simulink model "EGRVlv_DDSens"  (R2018a)
settings: configuration reference "cs_ert" (kept outside this file)
model workspace (MAT data in the model file):
  EGRVlv_DDSens_DT = 10
values from neighbouring files (symbols this model uses):
  EGRVlv_rAdapDiffPlausLgT_C = 20.0    [EGRVlv_DDSens.sldd]
  EGRVlv_rTransf_CUR : value not decoded    [EGRVlv_DDSens.sldd]
  EGRVlv_rTransf_CURX : value not decoded    [EGRVlv_DDSens.sldd]
  EGRVlv_tiMaxDefDeb_C = 200.0    [EGRVlv_DDSens.sldd]
  EGRVlv_tiMaxOKDeb_C = 200.0    [EGRVlv_DDSens.sldd]
  EGRVlv_tiMinDefDeb_C = 200.0    [EGRVlv_DDSens.sldd]
  EGRVlv_tiMinOKDeb_C = 200.0    [EGRVlv_DDSens.sldd]
  EGRVlv_tiPhysRngHiDefDeb_C = 200.0    [EGRVlv_DDSens.sldd]
  EGRVlv_tiPhysRngHiOKDeb_C = 200.0    [EGRVlv_DDSens.sldd]
  EGRVlv_tiPhysRngLoDefDeb_C = 200.0    [EGRVlv_DDSens.sldd]
  EGRVlv_tiPhysRngLoOKDeb_C = 200.0    [EGRVlv_DDSens.sldd]
  EGRVlv_uSRCMax_C = 4800.0    [EGRVlv_DDSens.sldd]
  EGRVlv_uSRCMin_C = 200.0    [EGRVlv_DDSens.sldd]
undefined symbols (not defined in the file or in its folder): CEngDsT_tTransf_CURX
libraries: sllib x4
settings Model: DataDictionary=EGRVlv_DDSens.sldd  Creator=zhoutinglin  LastModifiedBy=zhoutinglin

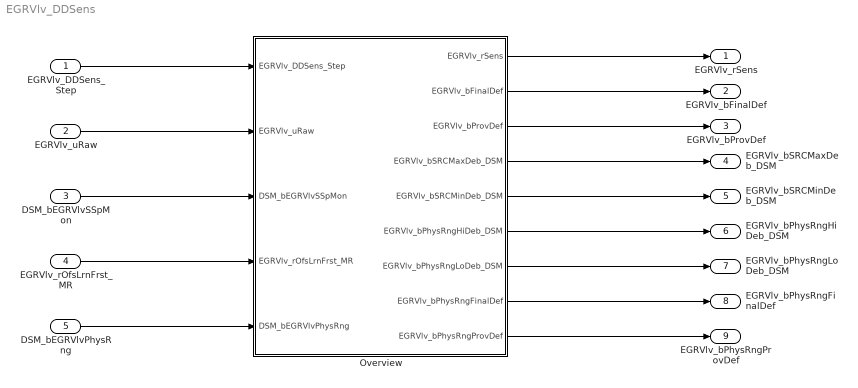
== system EGRVlv_DDSens ==
  EGRVlv_DDSens_Step : Inport  OutputFunctionCall=on
  EGRVlv_uRaw : Inport  Description=Raw voltage value of position sensor  Port=2  OutMin=0  OutMax=5000  OutDataTypeStr=Volt_mV  Unit=mv  PortDimensions=[1 1]
  DSM_bEGRVlvSSpMon : Inport  Description=Status of FId_EGRVlvSSpMon  Port=3  OutMin=0  OutMax=1  OutDataTypeStr=boolean  PortDimensions=[1 1]
  EGRVlv_rOfsLrnFrst_MR : Inport  Description=First learnt offset value read from EEPROM  Port=4  OutMin=-100  OutMax=100  OutDataTypeStr=DutyCycle  Unit=%  PortDimensions=[1 1]
  DSM_bEGRVlvPhysRng : Inport  Description=Status of FId_EGRVlvPhysRng  Port=5  OutMin=0  OutMax=1  OutDataTypeStr=boolean  PortDimensions=[1 1]
  Overview : Subsystem
  EGRVlv_rSens : Outport  Description=Sensed value of actuator position without error handling  OutMin=-100  OutMax=100  OutDataTypeStr=DutyCycle  Unit=%  PortDimensions=[1 1]
  EGRVlv_bFinalDef : Outport  Description=the final fault flag  Port=2  OutMin=0  OutMax=1  OutDataTypeStr=boolean  PortDimensions=[1 1]
  EGRVlv_bProvDef : Outport  Description=the fault flag for the moment  Port=3  OutMin=0  OutMax=1  OutDataTypeStr=boolean  PortDimensions=[1 1]
  EGRVlv_bSRCMaxDeb_DSM : Outport  Description=SRC High for EGR position sensor voltage  Port=4  OutMin=0  OutMax=1  OutDataTypeStr=boolean  PortDimensions=[1 1]
  EGRVlv_bSRCMinDeb_DSM : Outport  Description=SRC Low for EGR position sensor voltage  Port=5  OutMin=0  OutMax=1  OutDataTypeStr=boolean  PortDimensions=[1 1]
  EGRVlv_bPhysRngHiDeb_DSM : Outport  Description=Status of EGRVlv_bPhysRngHiDeb  Port=6  OutMin=0  OutMax=1  OutDataTypeStr=boolean  PortDimensions=[1 1]
  EGRVlv_bPhysRngLoDeb_DSM : Outport  Description=Status of EGRVlv_bPhysRngLoDeb  Port=7  OutMin=0  OutMax=1  OutDataTypeStr=boolean  PortDimensions=[1 1]
  EGRVlv_bPhysRngFinalDef : Outport  Description=Status Sensor of the EGR valve physical Signal range check finally defect  Port=8  OutMin=0  OutMax=1  OutDataTypeStr=boolean  PortDimensions=[1 1]
  EGRVlv_bPhysRngProvDef : Outport  Description=Status Sensor of the EGR valve physical Signal range check temporary defect  Port=9  OutMin=0  OutMax=1  OutDataTypeStr=boolean  PortDimensions=[1 1]
  wires:
  EGRVlv_DDSens_Step/1 -> Overview/1(EGRVlv_DDSens_Step)
  EGRVlv_uRaw/1 -> Overview/2(EGRVlv_uRaw)
  DSM_bEGRVlvSSpMon/1 -> Overview/3(DSM_bEGRVlvSSpMon)
  EGRVlv_rOfsLrnFrst_MR/1 -> Overview/4(EGRVlv_rOfsLrnFrst_MR)
  DSM_bEGRVlvPhysRng/1 -> Overview/5(DSM_bEGRVlvPhysRng)
  Overview/1(EGRVlv_rSens) -> EGRVlv_rSens/1
  Overview/2(EGRVlv_bFinalDef) -> EGRVlv_bFinalDef/1
  Overview/3(EGRVlv_bProvDef) -> EGRVlv_bProvDef/1
  Overview/4(EGRVlv_bSRCMaxDeb_DSM) -> EGRVlv_bSRCMaxDeb_DSM/1
  Overview/5(EGRVlv_bSRCMinDeb_DSM) -> EGRVlv_bSRCMinDeb_DSM/1
  Overview/6(EGRVlv_bPhysRngHiDeb_DSM) -> EGRVlv_bPhysRngHiDeb_DSM/1
  Overview/7(EGRVlv_bPhysRngLoDeb_DSM) -> EGRVlv_bPhysRngLoDeb_DSM/1
  Overview/8(EGRVlv_bPhysRngFinalDef) -> EGRVlv_bPhysRngFinalDef/1
  Overview/9(EGRVlv_bPhysRngProvDef) -> EGRVlv_bPhysRngProvDef/1

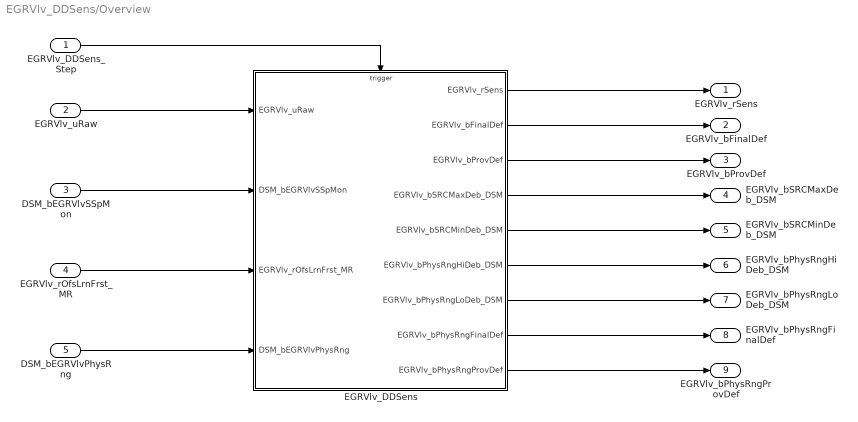
== system EGRVlv_DDSens/Overview ==
  EGRVlv_DDSens_Step : Inport
  EGRVlv_uRaw : Inport  Port=2
  DSM_bEGRVlvSSpMon : Inport  Port=3
  EGRVlv_rOfsLrnFrst_MR : Inport  Port=4
  DSM_bEGRVlvPhysRng : Inport  Port=5
  EGRVlv_DDSens : Subsystem
  EGRVlv_rSens : Outport
  EGRVlv_bFinalDef : Outport  Port=2
  EGRVlv_bProvDef : Outport  Port=3
  EGRVlv_bSRCMaxDeb_DSM : Outport  Port=4
  EGRVlv_bSRCMinDeb_DSM : Outport  Port=5
  EGRVlv_bPhysRngHiDeb_DSM : Outport  Port=6
  EGRVlv_bPhysRngLoDeb_DSM : Outport  Port=7
  EGRVlv_bPhysRngFinalDef : Outport  Port=8
  EGRVlv_bPhysRngProvDef : Outport  Port=9
  wires:
  EGRVlv_uRaw/1 -> EGRVlv_DDSens/1(EGRVlv_uRaw)
  DSM_bEGRVlvSSpMon/1 -> EGRVlv_DDSens/2(DSM_bEGRVlvSSpMon)
  EGRVlv_rOfsLrnFrst_MR/1 -> EGRVlv_DDSens/3(EGRVlv_rOfsLrnFrst_MR)
  DSM_bEGRVlvPhysRng/1 -> EGRVlv_DDSens/4(DSM_bEGRVlvPhysRng)
  EGRVlv_DDSens/1(EGRVlv_rSens) -> EGRVlv_rSens/1
  EGRVlv_DDSens/2(EGRVlv_bFinalDef) -> EGRVlv_bFinalDef/1
  EGRVlv_DDSens/3(EGRVlv_bProvDef) -> EGRVlv_bProvDef/1
  EGRVlv_DDSens/4(EGRVlv_bSRCMaxDeb_DSM) -> EGRVlv_bSRCMaxDeb_DSM/1
  EGRVlv_DDSens/5(EGRVlv_bSRCMinDeb_DSM) -> EGRVlv_bSRCMinDeb_DSM/1
  EGRVlv_DDSens/6(EGRVlv_bPhysRngHiDeb_DSM) -> EGRVlv_bPhysRngHiDeb_DSM/1
  EGRVlv_DDSens/7(EGRVlv_bPhysRngLoDeb_DSM) -> EGRVlv_bPhysRngLoDeb_DSM/1
  EGRVlv_DDSens/8(EGRVlv_bPhysRngFinalDef) -> EGRVlv_bPhysRngFinalDef/1
  EGRVlv_DDSens/9(EGRVlv_bPhysRngProvDef) -> EGRVlv_bPhysRngProvDef/1
  EGRVlv_DDSens_Step/1 -> EGRVlv_DDSens/Trigger

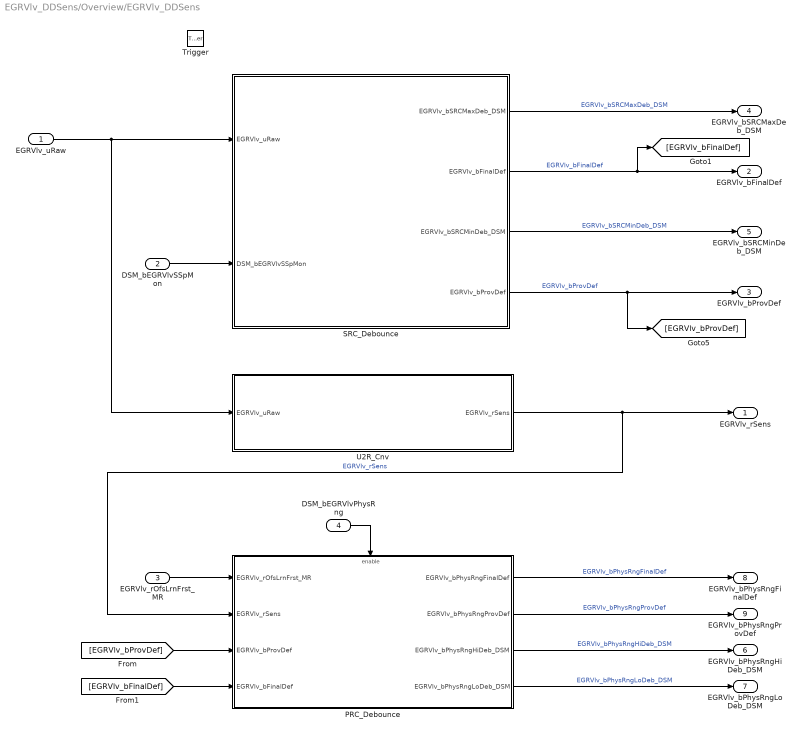
== system EGRVlv_DDSens/Overview/EGRVlv_DDSens ==
  EGRVlv_uRaw : Inport  Tag=mv
  DSM_bEGRVlvSSpMon : Inport  Port=2
  EGRVlv_rOfsLrnFrst_MR : Inport  Port=3
  DSM_bEGRVlvPhysRng : Inport  Port=4
  Trigger : TriggerPort  TriggerType=function-call  VariantControl=Variant  PortDimensions=1
  PRC_Debounce : Subsystem
  SRC_Debounce : Subsystem
  U2R_Cnv : Subsystem
  EGRVlv_rSens : Outport  Tag=%
  EGRVlv_bFinalDef : Outport  Port=2
  EGRVlv_bProvDef : Outport  Port=3
  EGRVlv_bSRCMaxDeb_DSM : Outport  Port=4
  EGRVlv_bSRCMinDeb_DSM : Outport  Port=5
  EGRVlv_bPhysRngHiDeb_DSM : Outport  Port=6
  EGRVlv_bPhysRngLoDeb_DSM : Outport  Port=7
  EGRVlv_bPhysRngFinalDef : Outport  Port=8
  EGRVlv_bPhysRngProvDef : Outport  Port=9
  wires:
  SRC_Debounce/2(EGRVlv_bFinalDef) -> EGRVlv_bFinalDef/1, [EGRVlv_bFinalDef]  "EGRVlv_bFinalDef"
  EGRVlv_uRaw/1 -> SRC_Debounce/1(EGRVlv_uRaw), U2R_Cnv/1(EGRVlv_uRaw)
  SRC_Debounce/4(EGRVlv_bProvDef) -> EGRVlv_bProvDef/1, [EGRVlv_bProvDef]  "EGRVlv_bProvDef"
  U2R_Cnv/1(EGRVlv_rSens) -> EGRVlv_rSens/1, PRC_Debounce/2(EGRVlv_rSens)  "EGRVlv_rSens"
  EGRVlv_rOfsLrnFrst_MR/1 -> PRC_Debounce/1(EGRVlv_rOfsLrnFrst_MR)
  [EGRVlv_bProvDef] -> PRC_Debounce/3(EGRVlv_bProvDef)
  [EGRVlv_bFinalDef] -> PRC_Debounce/4(EGRVlv_bFinalDef)
  DSM_bEGRVlvSSpMon/1 -> SRC_Debounce/2(DSM_bEGRVlvSSpMon)
  PRC_Debounce/1(EGRVlv_bPhysRngFinalDef) -> EGRVlv_bPhysRngFinalDef/1  "EGRVlv_bPhysRngFinalDef"
  PRC_Debounce/2(EGRVlv_bPhysRngProvDef) -> EGRVlv_bPhysRngProvDef/1  "EGRVlv_bPhysRngProvDef"
  PRC_Debounce/3(EGRVlv_bPhysRngHiDeb_DSM) -> EGRVlv_bPhysRngHiDeb_DSM/1  "EGRVlv_bPhysRngHiDeb_DSM"
  PRC_Debounce/4(EGRVlv_bPhysRngLoDeb_DSM) -> EGRVlv_bPhysRngLoDeb_DSM/1  "EGRVlv_bPhysRngLoDeb_DSM"
  SRC_Debounce/1(EGRVlv_bSRCMaxDeb_DSM) -> EGRVlv_bSRCMaxDeb_DSM/1  "EGRVlv_bSRCMaxDeb_DSM"
  SRC_Debounce/3(EGRVlv_bSRCMinDeb_DSM) -> EGRVlv_bSRCMinDeb_DSM/1  "EGRVlv_bSRCMinDeb_DSM"
  DSM_bEGRVlvPhysRng/1 -> PRC_Debounce/Enable

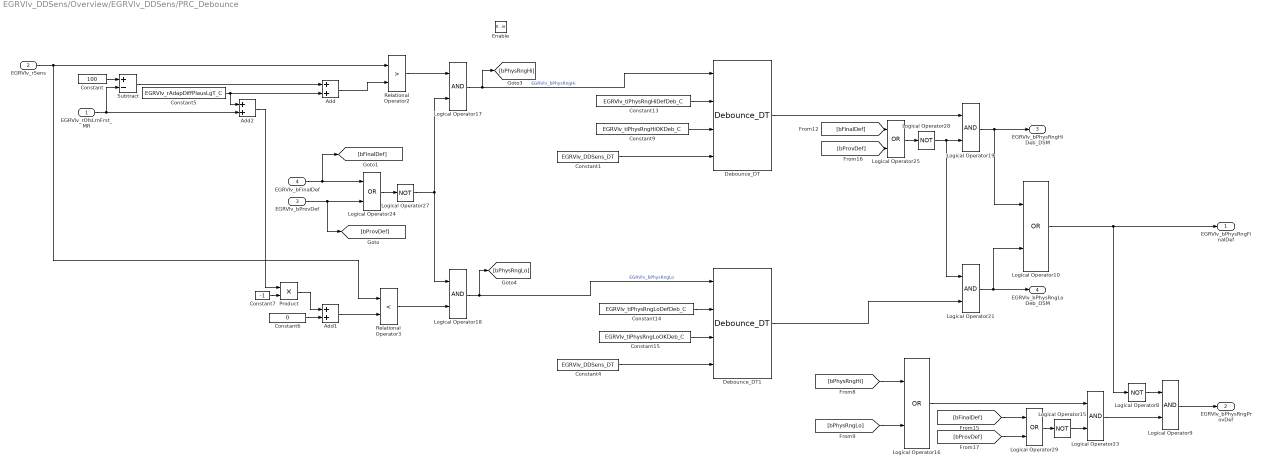
== system EGRVlv_DDSens/Overview/EGRVlv_DDSens/PRC_Debounce ==
  EGRVlv_rOfsLrnFrst_MR : Inport
  EGRVlv_rSens : Inport  Port=2
  EGRVlv_bProvDef : Inport  Port=3
  EGRVlv_bFinalDef : Inport  Port=4
  Enable : EnablePort
  Add : Sum  SaturateOnIntegerOverflow=on
  Add1 : Sum  SaturateOnIntegerOverflow=on  InputSameDT=on
  Add2 : Sum  SaturateOnIntegerOverflow=on
  Constant : Constant  Value=100  OutDataTypeStr=Inherit: Inherit via back propagation
  Constant1 : Constant  Value=EGRVlv_DDSens_DT  OutDataTypeStr=Inherit: Inherit via back propagation
  Constant13 : Constant  Value=EGRVlv_tiPhysRngHiDefDeb_C
  Constant14 : Constant  Value=EGRVlv_tiPhysRngLoDefDeb_C
  Constant15 : Constant  Value=EGRVlv_tiPhysRngLoOKDeb_C
  Constant4 : Constant  Value=EGRVlv_DDSens_DT  OutDataTypeStr=Inherit: Inherit via back propagation
  Constant5 : Constant  Value=EGRVlv_rAdapDiffPlausLgT_C
  Constant6 : Constant  Value=0  OutDataTypeStr=Inherit: Inherit via back propagation
  Constant7 : Constant  Value=-1  OutDataTypeStr=int8
  Constant9 : Constant  Value=EGRVlv_tiPhysRngHiOKDeb_C
  Debounce_DT : sllib/Debounce_DT
      settings: SourceProductName=sllib
  Debounce_DT1 : sllib/Debounce_DT
      settings: SourceProductName=sllib
  Logical Operator10 : Logic  Operator=OR  AllPortsSameDT=off  OutDataTypeStr=boolean
  Logical Operator{8,15,27..28} (4 alike) : Logic  Operator=NOT  AllPortsSameDT=off  OutDataTypeStr=boolean
  Logical Operator16 : Logic  Operator=OR  AllPortsSameDT=off  OutDataTypeStr=boolean
  Logical Operator{9,17..19,21,23} (6 alike) : Logic  AllPortsSameDT=off  OutDataTypeStr=boolean
  Logical Operator24 : Logic  Operator=OR  OutDataTypeStr=boolean
  Logical Operator25 : Logic  Operator=OR  OutDataTypeStr=boolean
  Logical Operator29 : Logic  Operator=OR  OutDataTypeStr=boolean
  Product : Product  OutDataTypeStr=Inherit: Inherit via back propagation  SaturateOnIntegerOverflow=on
  Relational Operator2 : RelationalOperator  Operator=>  OutDataTypeStr=boolean  RndMeth=Nearest  InputSameDT=on
  Relational Operator3 : RelationalOperator  Operator=<  OutDataTypeStr=boolean  RndMeth=Nearest  InputSameDT=on
  Subtract : Sum  Inputs=+-  SaturateOnIntegerOverflow=on
  EGRVlv_bPhysRngFinalDef : Outport  Tag=-  InitialOutput=0
  EGRVlv_bPhysRngProvDef : Outport  Tag=-  Port=2  InitialOutput=0
  EGRVlv_bPhysRngHiDeb_DSM : Outport  Tag=-  Port=3  InitialOutput=0
  EGRVlv_bPhysRngLoDeb_DSM : Outport  Tag=-  Port=4  InitialOutput=0
  wires:
  EGRVlv_rSens/1 -> Relational Operator2/1, Relational Operator3/1
  Constant15/1 -> Debounce_DT1/3
  Constant13/1 -> Debounce_DT/2
  Constant9/1 -> Debounce_DT/3
  Constant14/1 -> Debounce_DT1/2
  Constant1/1 -> Debounce_DT/4
  Constant4/1 -> Debounce_DT1/4
  Add/1 -> Relational Operator2/2
  Logical Operator17/1 -> Debounce_DT/1, [bPhysRngHi]  "EGRVlv_bPhysRngHi"
  Add1/1 -> Relational Operator3/2
  Logical Operator18/1 -> Debounce_DT1/1, [bPhysRngLo]  "EGRVlv_bPhysRngLo"
  Logical Operator19/1 -> Logical Operator10/1, EGRVlv_bPhysRngHiDeb_DSM/1
  Logical Operator21/1 -> EGRVlv_bPhysRngLoDeb_DSM/1, Logical Operator10/2
  [bPhysRngHi] -> Logical Operator16/1
  [bPhysRngLo] -> Logical Operator16/2
  Relational Operator2/1 -> Logical Operator17/1
  Logical Operator24/1 -> Logical Operator27/1
  Logical Operator25/1 -> Logical Operator28/1
  Logical Operator16/1 -> Logical Operator23/1
  Logical Operator15/1 -> Logical Operator23/2
  Relational Operator3/1 -> Logical Operator18/2
  EGRVlv_bFinalDef/1 -> [bFinalDef], Logical Operator24/1
  EGRVlv_bProvDef/1 -> Logical Operator24/2, [bProvDef]
  [bFinalDef] -> Logical Operator25/1
  [bProvDef] -> Logical Operator25/2
  Logical Operator27/1 -> Logical Operator17/2, Logical Operator18/1
  Logical Operator28/1 -> Logical Operator21/1, Logical Operator19/2
  [bFinalDef] -> Logical Operator29/1
  [bProvDef] -> Logical Operator29/2
  Logical Operator29/1 -> Logical Operator15/1
  Logical Operator10/1 -> EGRVlv_bPhysRngFinalDef/1, Logical Operator8/1
  Logical Operator8/1 -> Logical Operator9/1
  Logical Operator9/1 -> EGRVlv_bPhysRngProvDef/1
  Logical Operator23/1 -> Logical Operator9/2
  Constant/1 -> Subtract/1
  EGRVlv_rOfsLrnFrst_MR/1 -> Add2/2, Subtract/2
  Subtract/1 -> Add/1
  Constant5/1 -> Add/2, Add2/1
  Constant7/1 -> Product/2
  Constant6/1 -> Add1/2
  Product/1 -> Add1/1
  Add2/1 -> Product/1
  Debounce_DT/1 -> Logical Operator19/1
  Debounce_DT1/1 -> Logical Operator21/2

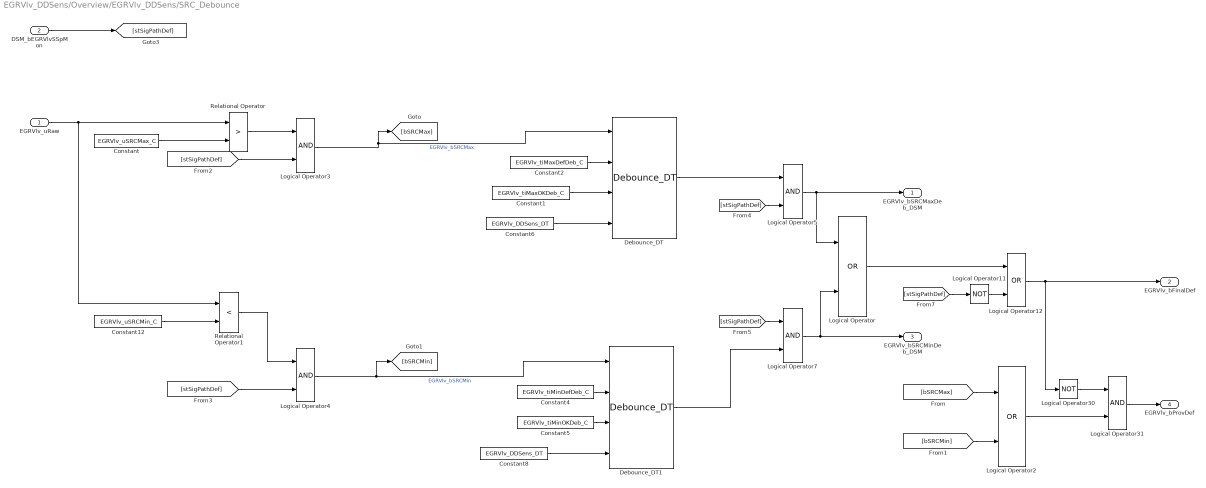
== system EGRVlv_DDSens/Overview/EGRVlv_DDSens/SRC_Debounce ==
  EGRVlv_uRaw : Inport  Tag=mv
  DSM_bEGRVlvSSpMon : Inport  Tag=-  Port=2
  Constant : Constant  Value=EGRVlv_uSRCMax_C
  Constant1 : Constant  Value=EGRVlv_tiMaxOKDeb_C
  Constant12 : Constant  Value=EGRVlv_uSRCMin_C
  Constant2 : Constant  Value=EGRVlv_tiMaxDefDeb_C
  Constant4 : Constant  Value=EGRVlv_tiMinDefDeb_C
  Constant5 : Constant  Value=EGRVlv_tiMinOKDeb_C
  Constant6 : Constant  Value=EGRVlv_DDSens_DT  OutDataTypeStr=Inherit: Inherit via back propagation
  Constant8 : Constant  Value=EGRVlv_DDSens_DT  OutDataTypeStr=Inherit: Inherit via back propagation
  Debounce_DT : sllib/Debounce_DT
      settings: SourceProductName=sllib
  Debounce_DT1 : sllib/Debounce_DT
      settings: SourceProductName=sllib
  Logical Operator : Logic  Operator=OR  AllPortsSameDT=off  OutDataTypeStr=boolean
  Logical Operator11 : Logic  Operator=NOT  AllPortsSameDT=off  OutDataTypeStr=boolean
  Logical Operator12 : Logic  Operator=OR  AllPortsSameDT=off  OutDataTypeStr=boolean
  Logical Operator2 : Logic  Operator=OR  AllPortsSameDT=off  OutDataTypeStr=boolean
  Logical Operator{3..5,7,31} (5 alike) : Logic  AllPortsSameDT=off  OutDataTypeStr=boolean
  Logical Operator30 : Logic  Operator=NOT  AllPortsSameDT=off  OutDataTypeStr=boolean
  Relational Operator : RelationalOperator  Operator=>  OutDataTypeStr=boolean  RndMeth=Nearest  InputSameDT=on
  Relational Operator1 : RelationalOperator  Operator=<  OutDataTypeStr=boolean  RndMeth=Nearest  InputSameDT=on
  EGRVlv_bSRCMaxDeb_DSM : Outport  Tag=-
  EGRVlv_bFinalDef : Outport  Tag=-  Port=2
  EGRVlv_bSRCMinDeb_DSM : Outport  Tag=-  Port=3
  EGRVlv_bProvDef : Outport  Tag=-  Port=4
  wires:
  Relational Operator1/1 -> Logical Operator4/1
  [stSigPathDef] -> Logical Operator4/2
  [stSigPathDef] -> Logical Operator5/2
  [stSigPathDef] -> Logical Operator7/1
  EGRVlv_uRaw/1 -> Relational Operator1/1, Relational Operator/1
  Logical Operator12/1 -> Logical Operator30/1, EGRVlv_bFinalDef/1
  Logical Operator30/1 -> Logical Operator31/1
  Logical Operator31/1 -> EGRVlv_bProvDef/1
  Logical Operator/1 -> Logical Operator12/1
  [stSigPathDef] -> Logical Operator11/1
  Logical Operator11/1 -> Logical Operator12/2
  Debounce_DT/1 -> Logical Operator5/1
  Constant4/1 -> Debounce_DT1/2
  Constant1/1 -> Debounce_DT/3
  Constant2/1 -> Debounce_DT/2
  Constant5/1 -> Debounce_DT1/3
  Constant6/1 -> Debounce_DT/4
  Constant8/1 -> Debounce_DT1/4
  Constant/1 -> Relational Operator/2
  Logical Operator3/1 -> Debounce_DT/1, [bSRCMax]  "EGRVlv_bSRCMax"
  Constant12/1 -> Relational Operator1/2
  Logical Operator4/1 -> Debounce_DT1/1, [bSRCMin]  "EGRVlv_bSRCMin"
  Logical Operator5/1 -> EGRVlv_bSRCMaxDeb_DSM/1, Logical Operator/1
  Logical Operator7/1 -> EGRVlv_bSRCMinDeb_DSM/1, Logical Operator/2
  [bSRCMax] -> Logical Operator2/1
  [bSRCMin] -> Logical Operator2/2
  DSM_bEGRVlvSSpMon/1 -> [stSigPathDef]
  Relational Operator/1 -> Logical Operator3/1
  [stSigPathDef] -> Logical Operator3/2
  Logical Operator2/1 -> Logical Operator31/2
  Debounce_DT1/1 -> Logical Operator7/2

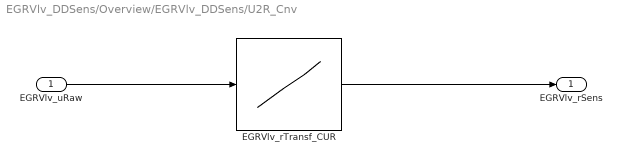
== system EGRVlv_DDSens/Overview/EGRVlv_DDSens/U2R_Cnv ==
  EGRVlv_uRaw : Inport  Tag=mv
  EGRVlv_rTransf_CUR : Lookup_n-D  DialogController=Simulink.DDGSource  NumberOfTableDimensions=1  BreakpointsForDimension1=EGRVlv_rTransf_CURX  BreakpointsForDimension2=CEngDsT_tTransf_CURX  IndexSearchMethod=Linear search  BeginIndexSearchUsingPreviousIndexResult=on  Table=EGRVlv_rTransf_CUR  TableDataTypeStr=Inherit: Inherit from 'Table data'  ExtrapMethod=Clip  UseLastTableValue=on  InternalRulePriority=Speed  OutDataTypeStr=Inherit: Inherit from 'Table data'  SaturateOnIntegerOverflow=on
  EGRVlv_rSens : Outport  Tag=%
  wires:
  EGRVlv_rTransf_CUR/1 -> EGRVlv_rSens/1
  EGRVlv_uRaw/1 -> EGRVlv_rTransf_CUR/1
